simulink model "test111"  (R2025b)
settings: Solver=ode113  StartTime=0.0  StopTime=10.0  RelTol=1e-8  AbsTol=1e-10
settings Model: Creator=mizula  LastModifiedBy=mizula

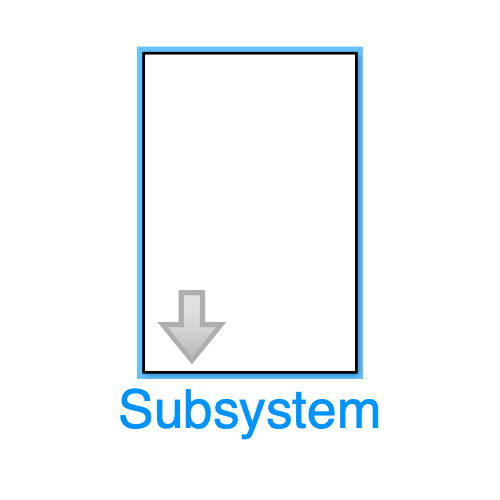
[thumbnail: Simulink's stored preview of the top-level diagram]
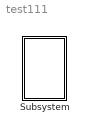
== system test111 ==
  Subsystem : Subsystem  mask{G=1, m1=1, m2=1, m3=1, x10=0.97000436, y10=0.24308753, vx10=0.466203685, vy10=-0.43236573, x20=0, y20=0, vx20=-0.93240737, vy20=0.86473146, x30=-0.97000436, y30=-0.24308753, vx30=0.466203685, vy30=-0.43236573}

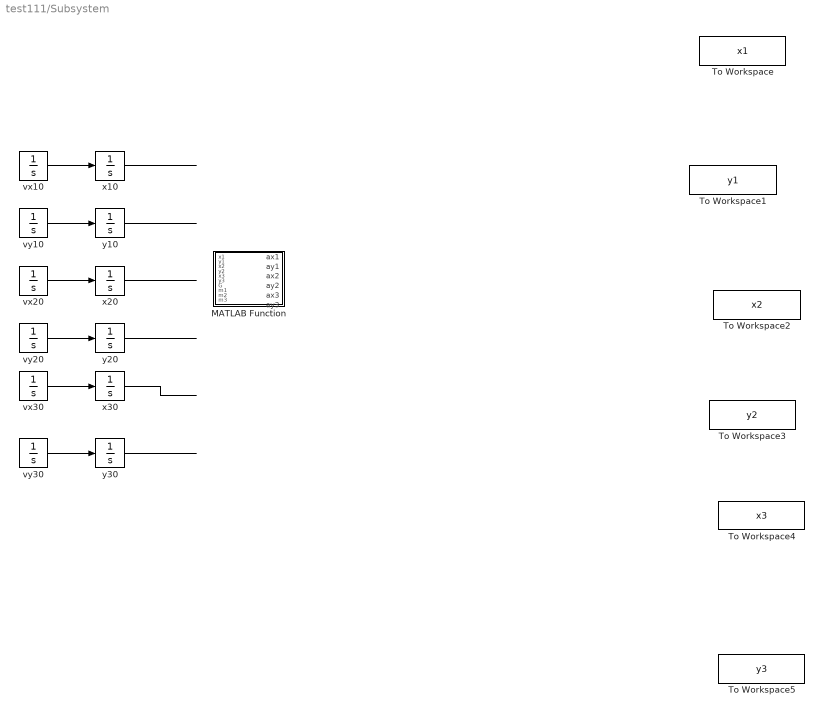
== system test111/Subsystem ==
  MATLAB Function : MATLAB Function  TreatAsAtomicUnit=on
  To Workspace : ToWorkspace  VariableName=x1  SaveFormat=Timeseries  SampleTime=-1
  To Workspace1 : ToWorkspace  VariableName=y1  SaveFormat=Timeseries  SampleTime=-1
  To Workspace2 : ToWorkspace  VariableName=x2  SaveFormat=Timeseries  SampleTime=-1
  To Workspace3 : ToWorkspace  VariableName=y2  SaveFormat=Timeseries  SampleTime=-1
  To Workspace4 : ToWorkspace  VariableName=x3  SaveFormat=Timeseries  SampleTime=-1
  To Workspace5 : ToWorkspace  VariableName=y3  SaveFormat=Timeseries  SampleTime=-1
  vx10 : Integrator  InitialCondition=vx10
  vx20 : Integrator  InitialCondition=vx20
  vx30 : Integrator  InitialCondition=vx30
  vy10 : Integrator  InitialCondition=vy10
  vy20 : Integrator  InitialCondition=vy20
  vy30 : Integrator  InitialCondition=vy30
  x10 : Integrator  InitialCondition=x10
  x20 : Integrator  InitialCondition=x20
  x30 : Integrator  InitialCondition=x30
  y10 : Integrator  InitialCondition=y10
  y20 : Integrator  InitialCondition=y20
  y30 : Integrator  InitialCondition=y30
  wires:
  vy20/1 -> y20/1
  vx30/1 -> x30/1
  ? -> vx10/1, To Workspace/1
  y20/1 -> ?
  ? -> To Workspace1/1, vy10/1
  ? -> To Workspace5/1, vy30/1
  x30/1 -> ?
  y10/1 -> ?
  x10/1 -> ?
  vx20/1 -> x20/1
  vx10/1 -> x10/1
  x20/1 -> ?
  y30/1 -> ?
  ? -> To Workspace4/1, vx30/1
  vy10/1 -> y10/1
  ? -> To Workspace2/1, vx20/1
  vy30/1 -> y30/1
  ? -> To Workspace3/1, vy20/1

== matlab function test111/Subsystem/MATLAB Function ==
  data: x1 input; ax1 output; y1 input; x2 input; y2 input; x3 input; y3 input; G input; m1 input; m2 input; m3 input; ay1 output; ax2 output; ay2 output; ax3 output; ay3 output
function [ax1, ay1, ax2, ay2, ax3, ay3] = fcn(x1,y1,x2,y2,x3,y3,G,m1,m2,m3)

r12 = ((x2-x1)^2 + (y2-y1)^2)^(3/2);
r13 = ((x3-x1)^2 + (y3-y1)^2)^(3/2);
r23 = ((x3-x2)^2 + (y3-y2)^2)^(3/2);

ax1 = G*m2*(x2-x1)/r12 + G*m3*(x3-x1)/r13;
ay1 = G*m2*(y2-y1)/r12 + G*m3*(y3-y1)/r13;

ax2 = G*m1*(x1-x2)/r12 + G*m3*(x3-x2)/r23;
ay2 = G*m1*(y1-y2)/r12 + G*m3*(y3-y2)/r23;

ax3 = G*m1*(x1-x3)/r13 + G*m2*(x2-x3)/r23;
ay3 = G*m1*(y1-y3)/r13 + G*m2*(y2-y3)/r23;

end
